simulink model "generic"  (Simulink 10.0)
settings: Solver=ode45  StartTime=0.0  StopTime=inf  RelTol=1e-3  EnableMultiTasking=on
libraries: CarMaker4SL x64, simulink x6
(part 3 of 3)

== system generic/CarMaker/VehicleControl/CreateBus VhclCtrl/Braking/Front Camera/While Iterator Subsystem3/If Action Subsystem2/If Action Subsystem2 ==
  Action Port : ActionPort  ActionPortLabel=if(u1>1)
  Constant : Constant  Commented=on  Value=30
  Constant1 : Constant  Commented=on  Value=5
  Write CM Dict : CarMaker4SL/Write CM Dict  Commented=on  xname=VC.Steer.AngAcc  xsync=off
  Write CM Dict1 : CarMaker4SL/Write CM Dict  Commented=on  xname=VC.Steer.Ang  xsync=off
  wires:
  Constant/1 -> Write CM Dict/1
  Constant1/1 -> Write CM Dict1/1

== system generic/CarMaker/VehicleControl/CreateBus VhclCtrl/Braking/Front Camera/While Iterator Subsystem3/If Action Subsystem2/If Action Subsystem4 ==
  Action Port : ActionPort  ActionPortLabel=else

== system generic/CarMaker/VehicleControl/CreateBus VhclCtrl/Braking/Subsystem6/While Iterator Subsystem/If Action Subsystem1/If Action Subsystem1 ==
  Action Port : ActionPort  ActionPortLabel=if(u1 ==1)
  Constant : Constant  Value=0
  Write CM Dict1 : CarMaker4SL/Write CM Dict  xname=VC.Gas  xsync=off
  wires:
  Constant/1 -> Write CM Dict1/1

== system generic/CarMaker/VehicleControl/CreateBus VhclCtrl/Braking/Subsystem6/While Iterator Subsystem/If Action Subsystem1/If Action Subsystem2 ==
  Action Port : ActionPort  ActionPortLabel=if(u1>1)
  Constant : Constant  Commented=on  Value=30
  Constant1 : Constant  Commented=on  Value=5
  Write CM Dict : CarMaker4SL/Write CM Dict  Commented=on  xname=VC.Steer.AngAcc  xsync=off
  Write CM Dict1 : CarMaker4SL/Write CM Dict  Commented=on  xname=VC.Steer.Ang  xsync=off
  wires:
  Constant/1 -> Write CM Dict/1
  Constant1/1 -> Write CM Dict1/1

== system generic/CarMaker/VehicleControl/CreateBus VhclCtrl/Braking/Subsystem6/While Iterator Subsystem/If Action Subsystem1/If Action Subsystem4 ==
  Action Port : ActionPort  ActionPortLabel=else
